simulink model "PEMFC500V_fmu"  (Simulink 10.2)
settings: Solver=FixedStepAuto  StartTime=0.0  StopTime=4900  FixedStep=0.001  RelTol=1e-6  EnableMultiTasking=on
undefined symbols (not defined in the file or in its folder): E0, Ncell
settings Model: Creator=podlam  LastModifiedBy=podlam
settings DataIOCC: LimitDataPoints=on  SignalLoggingName=sigsOut
settings OptimizationCC: InitFltsAndDblsToZero=on
settings DebuggingCC: SaveWithParameterizedLinksMsg=none  SignalResolutionControl=TryResolveAllWithWarning  MultiTaskDSMMsg=warning  MultiTaskCondExecSysMsg=none
settings HardwareCC: TargetUnknown=on
settings SFSimCC: SimUseLocalCustomCode=on  CustomCodeUndefinedFunction=FilterOut
settings RTWCC: RTWUseLocalCustomCode=on
settings GRTTargetCC: TargetFcnLib=ansi_tfl_tmw.mat
settings ConfigComp: CovExternalEMLEnable=on

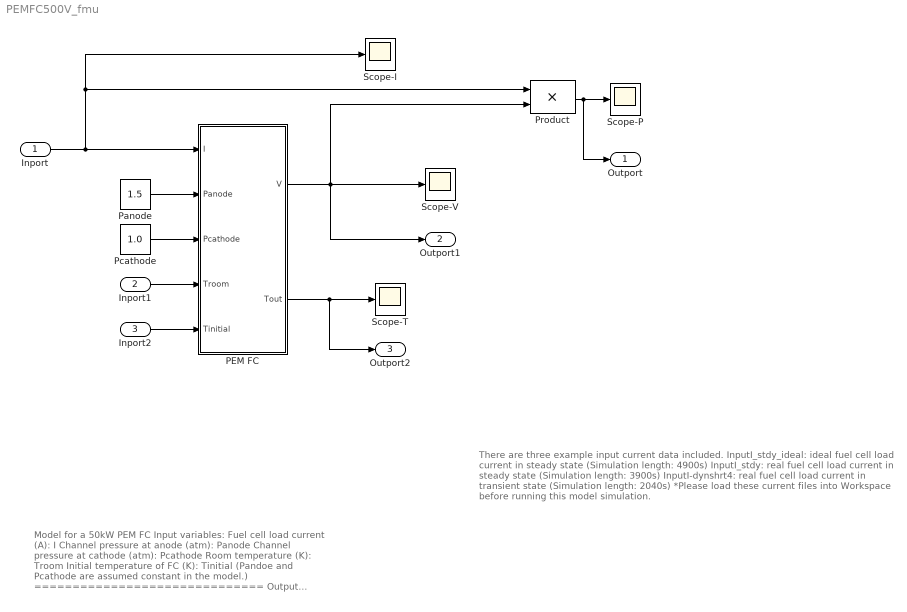
== system PEMFC500V_fmu ==
  note: Model for a 50kW PEM FC
      | Input variables:
      | Fuel cell load current (A): I
      | Channel pressure at anode (atm): Panode
      | Channel pressure at cathode (atm): Pcathode
      | Room temperature (K): Troom
      | Initial temperature of FC (K): Tinitial
      | (Pandoe and Pcathode are assumed constant in the model.)
      |
      | ==============================
      | Output variables:
      | Output terminal voltage (V): V
      | FC temperature (K): Tout
  note: There are three example input current data included.
      | InputI_stdy_ideal: ideal fuel cell load current in steady state (Simulation length: 4900s)
      | InputI_stdy: real fuel cell load current in steady state (Simulation length: 3900s)
      | InputI-dynshrt4: real fuel cell load current in transient state (Simulation length: 2040s)
      |
      | *Please load these current files into Workspace before running this model simulation.
  Inport : Inport
  Inport1 : Inport  Port=2
  Inport2 : Inport  Port=3
  PEM FC : Subsystem
  Panode : Constant  Value=1.5
  Pcathode : Constant  Value=1.0
  Product : Product  OutDataTypeStr=double  SaturateOnIntegerOverflow=on
  Scope-I : Scope
  Scope-P : Scope
  Scope-T : Scope
  Scope-V : Scope
  Outport : Outport
  Outport1 : Outport  Port=2
  Outport2 : Outport  Port=3
  wires:
  PEM FC/1(V) -> Product/2, Outport1/1, Scope-V/1
  Product/1 -> Outport/1, Scope-P/1
  Pcathode/1 -> PEM FC/3(Pcathode)
  Inport1/1 -> PEM FC/4(Troom)
  PEM FC/2(Tout) -> Outport2/1, Scope-T/1
  Inport2/1 -> PEM FC/5(Tinitial)
  Panode/1 -> PEM FC/2(Panode)
  Inport/1 -> Scope-I/1, Product/1, PEM FC/1(I)

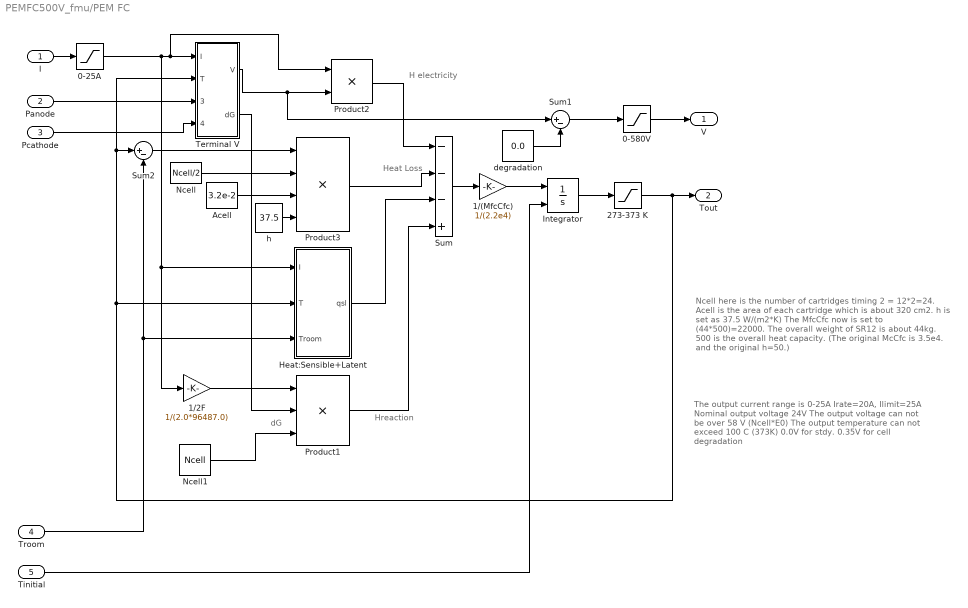
== system PEMFC500V_fmu/PEM FC ==
  note: Hreaction
  note: Heat Loss
  note: H electricity
  note: The output current range is 0-25A
      | Irate=20A, Ilimit=25A
      | Nominal output voltage 24V
      | The output voltage can not be over 58 V (Ncell*E0)
      | The output temperature can not exceed 100 C (373K)
      | 0.0V for stdy.
      | 0.35V for cell degradation
  note: dG
  note: Ncell here is the number of cartridges timing 2 = 12*2=24.
      | Acell is the area of each cartridge which is about 320 cm2.
      | h is set as 37.5 W/(m2*K)
      | The MfcCfc now is set to (44*500)=22000.
      | The overall weight of SR12 is about 44kg.
      | 500 is the overall heat capacity.
      | (The original McCfc is 3.5e4. and the original h=50.)
  I : Inport
  Panode : Inport  Port=2
  Pcathode : Inport  Port=3
  Troom : Inport  Port=4
  Tinitial : Inport  Port=5
  0-25A : Saturate  UpperLimit=25  LowerLimit=0
  0-580V : Saturate  UpperLimit=1500  LowerLimit=0
  1/(MfcCfc) : Gain  Gain=1/(2.2e4)  SaturateOnIntegerOverflow=on  OutDataTypeStr=Inherit: Same as input  ParamDataTypeStr=Inherit: Same as input
  1/2F : Gain  Gain=1/(2.0*96487.0)  SaturateOnIntegerOverflow=on  OutDataTypeStr=Inherit: Same as input  ParamDataTypeStr=Inherit: Same as input
  273-373 K : Saturate  UpperLimit=373.15  LowerLimit=273.15
  Acell : Constant  Value=3.2e-2
  Heat:Sensible+Latent : Subsystem
  Integrator : Integrator  InitialConditionSource=external
  Ncell : Constant  Value=Ncell/2
  Ncell1 : Constant  Value=Ncell
  Product1 : Product  Inputs=3  SaturateOnIntegerOverflow=on  OutDataTypeStr=Inherit: Same as first input
  Product2 : Product  SaturateOnIntegerOverflow=on  OutDataTypeStr=Inherit: Same as first input
  Product3 : Product  Inputs=4  SaturateOnIntegerOverflow=on  OutDataTypeStr=Inherit: Same as first input
  Sum : Sum  Inputs=---+  SaturateOnIntegerOverflow=on
  Sum1 : Sum  Inputs=|+-  SaturateOnIntegerOverflow=on
  Sum2 : Sum  Inputs=|+-  SaturateOnIntegerOverflow=on
  Terminal V : Subsystem
  degradation : Constant  Value=0.0
  h : Constant  Value=37.5
  V : Outport
  Tout : Outport  Port=2
  wires:
  I/1 -> 0-25A/1
  1/(MfcCfc)/1 -> Integrator/1
  1/2F/1 -> Product1/1
  Product2/1 -> Sum/1
  Product3/1 -> Sum/2
  Sum/1 -> 1/(MfcCfc)/1
  Troom/1 -> Sum2/2, Heat:Sensible+Latent/3(Troom)
  h/1 -> Product3/4
  Acell/1 -> Product3/3
  Ncell/1 -> Product3/2
  Sum2/1 -> Product3/1
  Ncell1/1 -> Product1/3
  Integrator/1 -> 273-373 K/1
  273-373 K/1 -> Tout/1, Sum2/1, Terminal V/2(T), Heat:Sensible+Latent/2(T)
  Panode/1 -> Terminal V/3(Panode)
  Pcathode/1 -> Terminal V/4(Pcathode)
  Terminal V/1(V) -> Product2/2, Sum1/1
  Product1/1 -> Sum/4
  Heat:Sensible+Latent/1(qsl) -> Sum/3
  0-25A/1 -> Product2/1, Terminal V/1(I), 1/2F/1, Heat:Sensible+Latent/1(I)
  Terminal V/2(dG) -> Product1/2
  0-580V/1 -> V/1
  Sum1/1 -> 0-580V/1
  degradation/1 -> Sum1/2
  Tinitial/1 -> Integrator/2

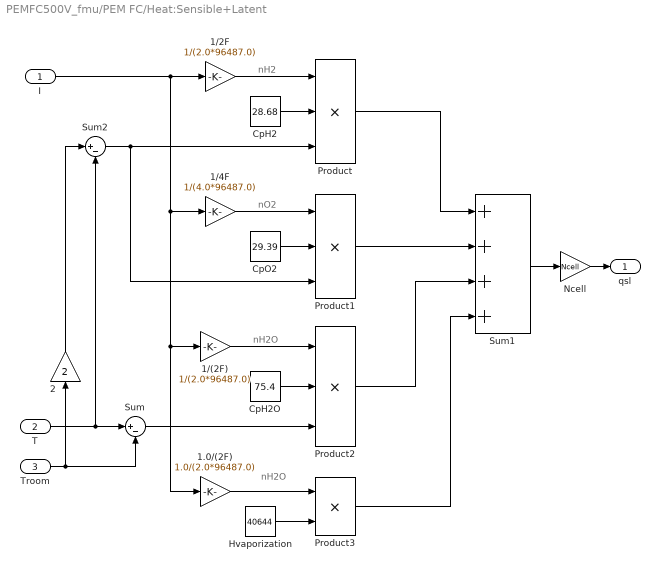
== system PEMFC500V_fmu/PEM FC/Heat:Sensible+Latent ==
  note: nH2
  note: nO2
  note: nH2O
  note: nH2O
  I : Inport
  T : Inport  Port=2
  Troom : Inport  Port=3
  1.0/(2F) : Gain  Gain=1.0/(2.0*96487.0)  SaturateOnIntegerOverflow=on  OutDataTypeStr=Inherit: Same as input  ParamDataTypeStr=Inherit: Same as input
  1/(2F) : Gain  Gain=1/(2.0*96487.0)  SaturateOnIntegerOverflow=on  OutDataTypeStr=Inherit: Same as input  ParamDataTypeStr=Inherit: Same as input
  1/2F : Gain  Gain=1/(2.0*96487.0)  SaturateOnIntegerOverflow=on  OutDataTypeStr=Inherit: Same as input  ParamDataTypeStr=Inherit: Same as input
  1/4F : Gain  Gain=1/(4.0*96487.0)  SaturateOnIntegerOverflow=on  OutDataTypeStr=Inherit: Same as input  ParamDataTypeStr=Inherit: Same as input
  2 : Gain  Gain=2  SaturateOnIntegerOverflow=on  OutDataTypeStr=Inherit: Same as input  ParamDataTypeStr=Inherit: Same as input
  CpH2 : Constant  Value=28.68
  CpH2O : Constant  Value=75.4
  CpO2 : Constant  Value=29.39
  Hvaporization : Constant  Value=40644
  Ncell : Gain  Gain=Ncell  SaturateOnIntegerOverflow=on  OutDataTypeStr=Inherit: Same as input  ParamDataTypeStr=Inherit: Same as input
  Product : Product  Inputs=3  SaturateOnIntegerOverflow=on  OutDataTypeStr=Inherit: Same as first input
  Product1 : Product  Inputs=3  SaturateOnIntegerOverflow=on  OutDataTypeStr=Inherit: Same as first input
  Product2 : Product  Inputs=3  SaturateOnIntegerOverflow=on  OutDataTypeStr=Inherit: Same as first input
  Product3 : Product  SaturateOnIntegerOverflow=on  OutDataTypeStr=Inherit: Same as first input
  Sum : Sum  Inputs=|+-  SaturateOnIntegerOverflow=on
  Sum1 : Sum  Inputs=++++  SaturateOnIntegerOverflow=on
  Sum2 : Sum  Inputs=|+-  SaturateOnIntegerOverflow=on
  qsl : Outport
  wires:
  I/1 -> 1.0/(2F)/1, 1/(2F)/1, 1/4F/1, 1/2F/1
  T/1 -> Sum/1, Sum2/2
  Troom/1 -> Sum/2, 2/1
  1/2F/1 -> Product/1
  CpH2/1 -> Product/2
  1/4F/1 -> Product1/1
  1/(2F)/1 -> Product2/1
  CpH2O/1 -> Product2/2
  1.0/(2F)/1 -> Product3/1
  Hvaporization/1 -> Product3/2
  Sum/1 -> Product2/3
  CpO2/1 -> Product1/2
  Product/1 -> Sum1/1
  Product1/1 -> Sum1/2
  Product2/1 -> Sum1/3
  Product3/1 -> Sum1/4
  Sum1/1 -> Ncell/1
  Ncell/1 -> qsl/1
  2/1 -> Sum2/1
  Sum2/1 -> Product/3, Product1/3

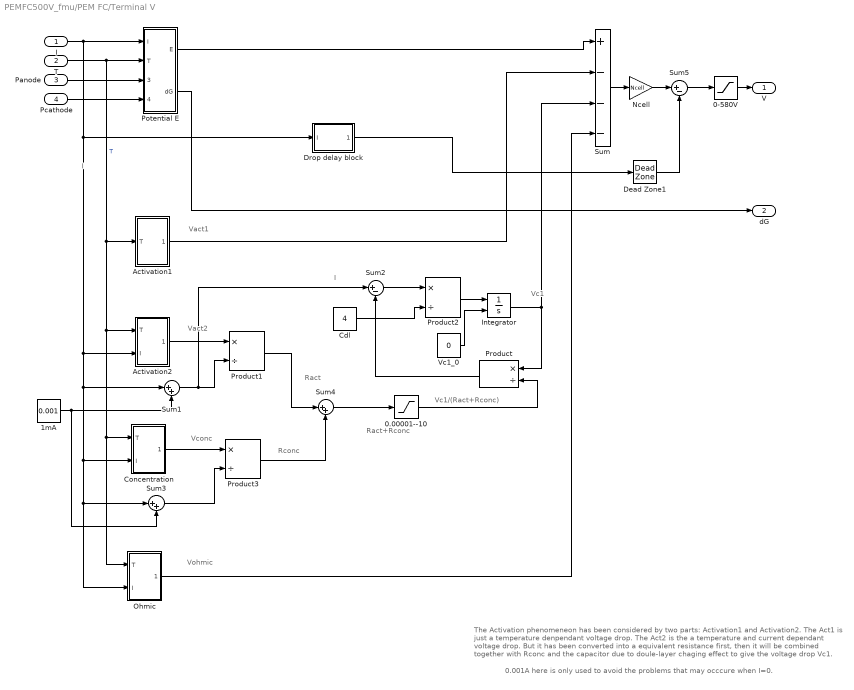
== system PEMFC500V_fmu/PEM FC/Terminal V ==
  note: I
  note: Ract
  note: Rconc
  note: Vc1
  note: Ract+Rconc
  note: Vc1/(Ract+Rconc)
  note: Vohmic
  note: Vact2
  note: Vconc
  note: I
  note: Vact1
  note: 0.001A here is only used to avoid the problems that may occcure when I=0.
  note: The Activation phenomeneon has been considered by two parts: Activation1 and Activation2.
      | The Act1 is just a temperature denpendant voltage drop.
      | The Act2 is the a temperature and current dependant voltage drop.
      | But it has been converted into a equivalent resistance first, then it will be combined together with Rconc
      | and the capacitor due to doule-layer chaging effect to give the voltage drop Vc1.
  I : Inport
  T : Inport  Port=2
  Panode : Inport  Port=3
  Pcathode : Inport  Port=4
  0-580V : Saturate  UpperLimit=1500  LowerLimit=0
  0.00001--10 : Saturate  UpperLimit=10  LowerLimit=0.00001
  1mA : Constant  Value=0.001
  Activation1 : Subsystem
  Activation2 : Subsystem
  Cdl : Constant  Value=4
  Concentration : Subsystem
  Dead Zone1 : DeadZone  LowerValue=-0.05  UpperValue=0.05  SaturateOnIntegerOverflow=on
  "Drop delay block " : Subsystem
  Integrator : Integrator  InitialConditionSource=external
  Ncell : Gain  Gain=Ncell  SaturateOnIntegerOverflow=on  OutDataTypeStr=Inherit: Same as input  ParamDataTypeStr=Inherit: Same as input
  Ohmic : Subsystem
  Potential E : Subsystem
  Product{,1..3} (4 alike) : Product  Inputs=*/  SaturateOnIntegerOverflow=on  OutDataTypeStr=Inherit: Same as first input
  Sum : Sum  Inputs=+---  SaturateOnIntegerOverflow=on
  Sum1 : Sum  Inputs=|++  SaturateOnIntegerOverflow=on
  Sum2 : Sum  Inputs=|+-  SaturateOnIntegerOverflow=on
  Sum3 : Sum  Inputs=|++  SaturateOnIntegerOverflow=on
  Sum4 : Sum  Inputs=|++  SaturateOnIntegerOverflow=on
  Sum5 : Sum  Inputs=|+-  SaturateOnIntegerOverflow=on
  Vc1_0 : Constant  Value=0
  V : Outport
  dG : Outport  Port=2
  wires:
  I/1 -> Potential E/1(I), "Drop delay block "/1(I), Activation2/2(I), Sum1/1, Concentration/2(I), Sum3/1, Ohmic/2(I)
  T/1 -> Potential E/2(T), Activation2/1(T), Concentration/1(T), Ohmic/1(T), Activation1/1(T)  "T"
  Potential E/1(E) -> Sum/1
  Sum/1 -> Ncell/1
  Panode/1 -> Potential E/3(Panode)
  Pcathode/1 -> Potential E/4(Pcathode)
  Potential E/2(dG) -> dG/1
  Activation2/1(Act2) -> Product1/1
  1mA/1 -> Sum1/2, Sum3/2
  Sum1/1 -> Product1/2, Sum2/1
  Integrator/1 -> Product/1, Sum/3
  Sum4/1 -> 0.00001--10/1
  Product/1 -> Sum2/2
  Sum2/1 -> Product2/1
  Cdl/1 -> Product2/2
  Product2/1 -> Integrator/1
  Vc1_0/1 -> Integrator/2
  Concentration/1(Conc) -> Product3/1
  Sum3/1 -> Product3/2
  Product3/1 -> Sum4/2
  Product1/1 -> Sum4/1
  Ohmic/1(Ohmic) -> Sum/4
  0.00001--10/1 -> Product/2
  0-580V/1 -> V/1
  Ncell/1 -> Sum5/1
  Sum5/1 -> 0-580V/1
  Dead Zone1/1 -> Sum5/2
  "Drop delay block "/1(Vdyn_d) -> Dead Zone1/1
  Activation1/1(Act1) -> Sum/2

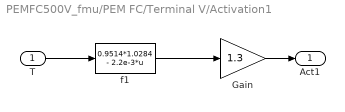
== system PEMFC500V_fmu/PEM FC/Terminal V/Activation1 ==
  T : Inport
  Gain : Gain  Gain=1.3  SaturateOnIntegerOverflow=on  OutDataTypeStr=Inherit: Same as input  ParamDataTypeStr=Inherit: Same as input
  f1 : Fcn  Expr=0.9514*1.0284 - 2.2e-3*u
  Act1 : Outport
  wires:
  f1/1 -> Gain/1
  T/1 -> f1/1
  Gain/1 -> Act1/1

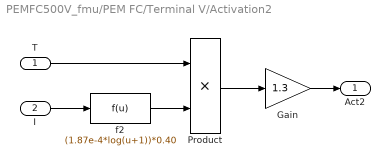
== system PEMFC500V_fmu/PEM FC/Terminal V/Activation2 ==
  T : Inport
  I : Inport  Port=2
  Gain : Gain  Gain=1.3  SaturateOnIntegerOverflow=on  OutDataTypeStr=Inherit: Same as input  ParamDataTypeStr=Inherit: Same as input
  Product : Product  SaturateOnIntegerOverflow=on  OutDataTypeStr=Inherit: Same as first input
  f2 : Fcn  Expr=(1.87e-4*log(u+1))*0.40
  Act2 : Outport
  wires:
  f2/1 -> Product/2
  Product/1 -> Gain/1
  T/1 -> Product/1
  I/1 -> f2/1
  Gain/1 -> Act2/1

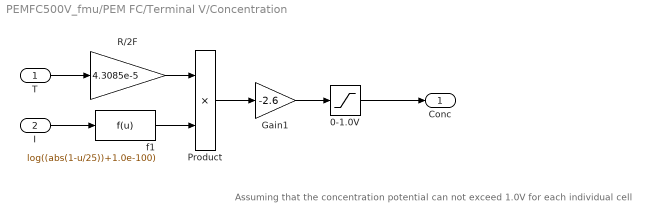
== system PEMFC500V_fmu/PEM FC/Terminal V/Concentration ==
  note: Assuming that the concentration potential can not exceed 1.0V for each individual cell
  T : Inport
  I : Inport  Port=2
  0-1.0V : Saturate  UpperLimit=1.0  LowerLimit=0
  Gain1 : Gain  Gain=-2.6  SaturateOnIntegerOverflow=on  OutDataTypeStr=Inherit: Same as input  ParamDataTypeStr=Inherit: Same as input
  Product : Product  SaturateOnIntegerOverflow=on  OutDataTypeStr=Inherit: Same as first input
  R/2F : Gain  Gain=4.3085e-5  SaturateOnIntegerOverflow=on  OutDataTypeStr=Inherit: Same as input  ParamDataTypeStr=Inherit: Same as input
  f1 : Fcn  Expr=log((abs(1-u/25))+1.0e-100)
  Conc : Outport
  wires:
  R/2F/1 -> Product/1
  T/1 -> R/2F/1
  Product/1 -> Gain1/1
  I/1 -> f1/1
  f1/1 -> Product/2
  0-1.0V/1 -> Conc/1
  Gain1/1 -> 0-1.0V/1

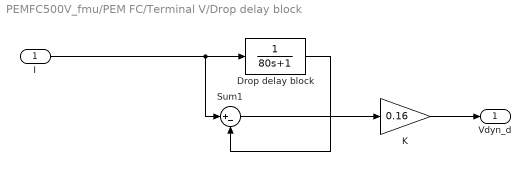
== system PEMFC500V_fmu/PEM FC/Terminal V/Drop delay block  ==
  I : Inport
  Drop delay block : TransferFcn  Denominator=[80,1]
  K : Gain  Gain=0.16  SaturateOnIntegerOverflow=on  OutDataTypeStr=Inherit: Same as input  ParamDataTypeStr=Inherit: Same as input
  Sum1 : Sum  Inputs=|+-  SaturateOnIntegerOverflow=on
  Vdyn_d : Outport
  wires:
  Drop delay block/1 -> Sum1/2
  Sum1/1 -> K/1
  K/1 -> Vdyn_d/1
  I/1 -> Sum1/1, Drop delay block/1

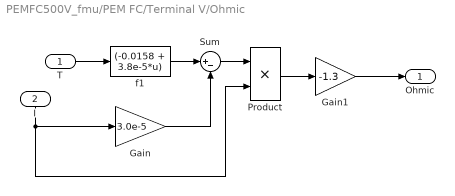
== system PEMFC500V_fmu/PEM FC/Terminal V/Ohmic ==
  T : Inport
  I : Inport  Port=2
  Gain : Gain  Gain=3.0e-5  SaturateOnIntegerOverflow=on  OutDataTypeStr=Inherit: Same as input  ParamDataTypeStr=Inherit: Same as input
  Gain1 : Gain  Gain=-1.3  SaturateOnIntegerOverflow=on  OutDataTypeStr=Inherit: Same as input  ParamDataTypeStr=Inherit: Same as input
  Product : Product  SaturateOnIntegerOverflow=on  OutDataTypeStr=Inherit: Same as first input
  Sum : Sum  Inputs=|+-  SaturateOnIntegerOverflow=on
  f1 : Fcn  Expr=(-0.0158 + 3.8e-5*u)
  Ohmic : Outport
  wires:
  f1/1 -> Sum/1
  Gain/1 -> Sum/2
  Sum/1 -> Product/1
  T/1 -> f1/1
  I/1 -> Gain/1, Product/2
  Product/1 -> Gain1/1
  Gain1/1 -> Ohmic/1

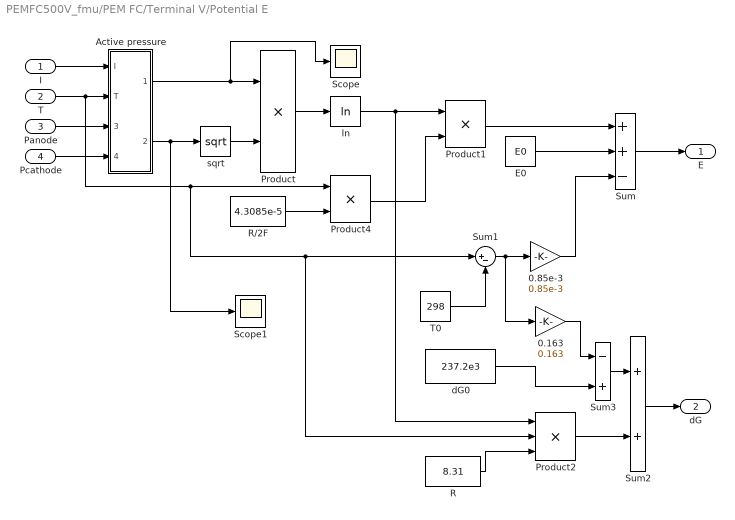
== system PEMFC500V_fmu/PEM FC/Terminal V/Potential E ==
  I : Inport
  T : Inport  Port=2
  Panode : Inport  Port=3
  Pcathode : Inport  Port=4
  0.163 : Gain  Gain=0.163  SaturateOnIntegerOverflow=on  OutDataTypeStr=Inherit: Same as input  ParamDataTypeStr=Inherit: Same as input
  0.85e-3 : Gain  Gain=0.85e-3  SaturateOnIntegerOverflow=on  OutDataTypeStr=Inherit: Same as input  ParamDataTypeStr=Inherit: Same as input
  Active pressure : Subsystem
  E0 : Constant  Value=E0
  Product : Product  SaturateOnIntegerOverflow=on  OutDataTypeStr=Inherit: Same as first input
  Product1 : Product  SaturateOnIntegerOverflow=on  OutDataTypeStr=Inherit: Same as first input
  Product2 : Product  Inputs=3  SaturateOnIntegerOverflow=on  OutDataTypeStr=Inherit: Same as first input
  Product4 : Product  SaturateOnIntegerOverflow=on  OutDataTypeStr=Inherit: Same as first input
  R : Constant  Value=8.31
  R/2F : Constant  Value=4.3085e-5
  Scope : Scope
  Scope1 : Scope
  Sum : Sum  Inputs=++-  SaturateOnIntegerOverflow=on
  Sum1 : Sum  Inputs=|+-  SaturateOnIntegerOverflow=on
  Sum2 : Sum  SaturateOnIntegerOverflow=on
  Sum3 : Sum  Inputs=-+  SaturateOnIntegerOverflow=on
  T0 : Constant  Value=298
  dG0 : Constant  Value=237.2e3
  ln : Math  Operator=log  SignedPower=on  SaturateOnIntegerOverflow=on
  sqrt : Math  Operator=sqrt  SignedPower=on  SaturateOnIntegerOverflow=on
  E : Outport
  dG : Outport  Port=2
  wires:
  I/1 -> Active pressure/1(I)
  Active pressure/1(PH2) -> Product/1, Scope/1
  T/1 -> Product4/1, Sum1/1, Product2/2, Active pressure/2(T)
  Active pressure/2(PO2) -> sqrt/1, Scope1/1
  sqrt/1 -> Product/2
  Product/1 -> ln/1
  R/2F/1 -> Product4/2
  ln/1 -> Product1/1, Product2/1
  Product4/1 -> Product1/2
  Product1/1 -> Sum/1
  Sum/1 -> E/1
  Panode/1 -> Active pressure/3(Panode)
  Pcathode/1 -> Active pressure/4(Pcathode)
  T0/1 -> Sum1/2
  E0/1 -> Sum/2
  Sum1/1 -> 0.85e-3/1, 0.163/1
  0.85e-3/1 -> Sum/3
  Sum2/1 -> dG/1
  R/1 -> Product2/3
  Product2/1 -> Sum2/2
  dG0/1 -> Sum3/2
  0.163/1 -> Sum3/1
  Sum3/1 -> Sum2/1

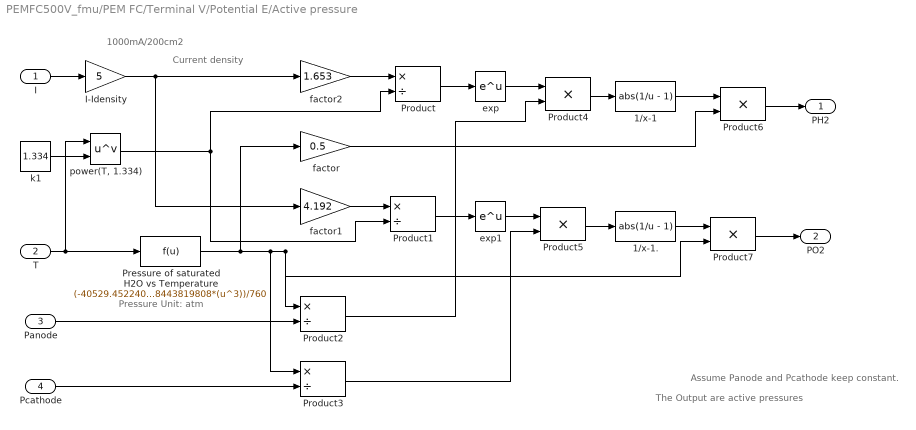
== system PEMFC500V_fmu/PEM FC/Terminal V/Potential E/Active pressure ==
  note: Current density
  note: Pressure Unit: atm
  note: 1000mA/200cm2
  note: Assume Panode and Pcathode keep constant.
  note: The Output are active pressures
  I : Inport
  T : Inport  Port=2
  Panode : Inport  Port=3
  Pcathode : Inport  Port=4
  1/x-1 : Fcn  Expr=abs(1/u - 1)
  1/x-1. : Fcn  Expr=abs(1/u - 1)
  I-Idensity : Gain  Gain=5  SaturateOnIntegerOverflow=on  OutDataTypeStr=Inherit: Same as input  ParamDataTypeStr=Inherit: Same as input
  Pressure of saturated H2O vs Temperature : Fcn  Expr=(-40529.4522405347 + 401.94033912153*u-1.33430273535993*(u^2) + 0.00148378443819808*(u^3))/760
  Product{,1..3} (4 alike) : Product  Inputs=*/  SaturateOnIntegerOverflow=on  OutDataTypeStr=Inherit: Same as first input
  Product{4..7} (4 alike) : Product  SaturateOnIntegerOverflow=on  OutDataTypeStr=Inherit: Same as first input
  exp : Math  SignedPower=on  SaturateOnIntegerOverflow=on
  exp1 : Math  SignedPower=on  SaturateOnIntegerOverflow=on
  factor : Gain  Gain=0.5  SaturateOnIntegerOverflow=on  OutDataTypeStr=Inherit: Same as input  ParamDataTypeStr=Inherit: Same as input
  factor1 : Gain  Gain=4.192  SaturateOnIntegerOverflow=on  OutDataTypeStr=Inherit: Same as input  ParamDataTypeStr=Inherit: Same as input
  factor2 : Gain  Gain=1.653  SaturateOnIntegerOverflow=on  OutDataTypeStr=Inherit: Same as input  ParamDataTypeStr=Inherit: Same as input
  k1 : Constant  Value=1.334
  "power(T, 1.334)" : Math  Operator=pow  SignedPower=on  SaturateOnIntegerOverflow=on
  PH2 : Outport
  PO2 : Outport  Port=2
  wires:
  T/1 -> "power(T, 1.334)"/1, Pressure of saturated H2O vs Temperature/1
  Pressure of saturated H2O vs Temperature/1 -> factor/1, Product3/1, Product2/1, Product7/2
  I/1 -> I-Idensity/1
  k1/1 -> "power(T, 1.334)"/2
  "power(T, 1.334)"/1 -> Product/2, Product1/2
  factor2/1 -> Product/1
  factor1/1 -> Product1/1
  Product/1 -> exp/1
  Product1/1 -> exp1/1
  Panode/1 -> Product2/2
  Pcathode/1 -> Product3/2
  Product2/1 -> Product4/2
  exp/1 -> Product4/1
  exp1/1 -> Product5/1
  Product3/1 -> Product5/2
  Product4/1 -> 1/x-1/1
  Product5/1 -> 1/x-1./1
  1/x-1/1 -> Product6/1
  factor/1 -> Product6/2
  1/x-1./1 -> Product7/1
  Product6/1 -> PH2/1
  Product7/1 -> PO2/1
  I-Idensity/1 -> factor1/1, factor2/1
